simulink model "unicycle_control_template_R2018a"  (R2021a)
settings: Solver=ode23  StartTime=0.0  StopTime=100  RelTol=1e-5
PreLoadFcn:
  | % initialize variables
  | initializeUnicycleModel;
undefined symbols (not defined in the file or in its folder): unicycle
settings Model: Creator=beniamino  LastModifiedBy=pasqu
settings SolverCC: ZeroCrossAlgorithm=Adaptive  AlgebraicLoopSolver=TrustRegion
settings DataIOCC: InitialState=cartesianInitialStates  SaveFormat=StructureWithTime  SaveOutput=off  SignalLogging=off  DSMLogging=off  SaveTime=off  ReturnWorkspaceOutputs=off
settings DebuggingCC: IgnoredZcDiagnostic=none  ArithmeticOperatorsInVariantConditions=warning
settings SFSimCC: CustomCodeUndefinedFunction=UseInterfaceOnly

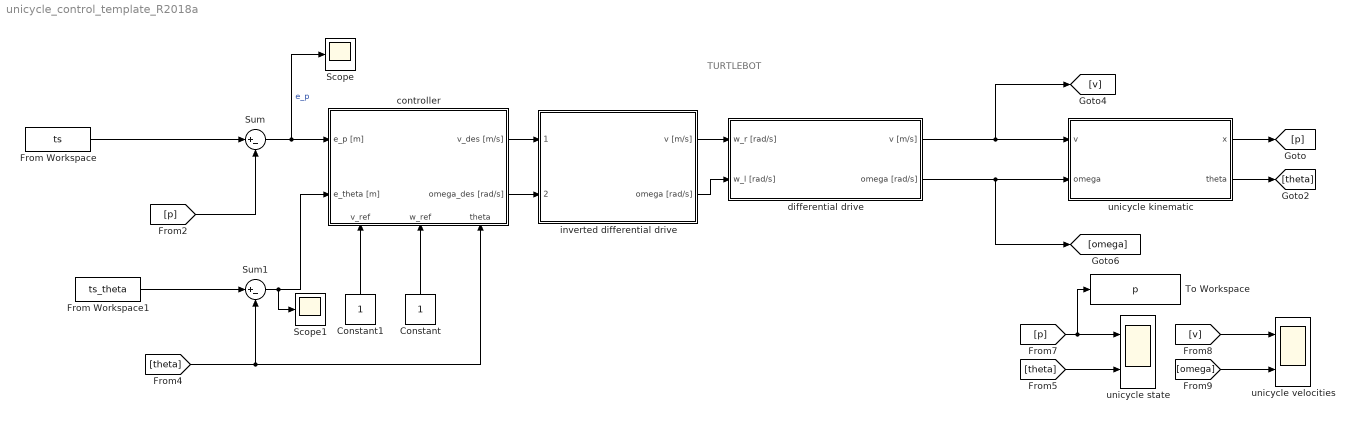
== system unicycle_control_template_R2018a ==
  note: TURTLEBOT
  Constant : Constant
  Constant1 : Constant
  From Workspace : FromWorkspace  VariableName=ts  OutputAfterFinalValue=Holding final value
  From Workspace1 : FromWorkspace  VariableName=ts_theta  OutputAfterFinalValue=Holding final value
  Scope : Scope
  Scope1 : Scope
  Sum : Sum  Inputs=|+-
  Sum1 : Sum  Inputs=|+-
  To Workspace : ToWorkspace  VariableName=p  SaveFormat=Structure With Time  SampleTime=-1
  controller : Subsystem
      settings: PortSchema="{\"entries\":[{\"content\":{\"sides\":[{\"content\":{\"connectorIds\":[\"In1\",\"In2\"]},\"type\":\"ConnectorPlacement.EquallySpacedRectSide\",\"uuid\":\"3f4c2626-0e3e-4d8a-88ac-bb46b09b9e2c\"},{\"content\":{\"connectorIds\":[\"Out1\",\"Out2\"],\"side\":\"RIGHT\"},\"type\":\"ConnectorPlacement.EquallySpacedRectSide\",\"uuid\":\"0c477789-f901-42f2-a0ef-9ff1b1969988\"},{\"content\":{\"connectorIds\":[],\"side\":\"TOP\"},\"type\":\"ConnectorPlacement.EquallySpacedRectSide\",\"uuid\":\"69e4ed00-4175-4f37-9b31-402b95ddf552\"},{\"content\":{\"connectorIds\":[\"In3\",\"In4\",\"In5\"],\"side\":\"BOTTOM\"},\"type\":\"ConnectorPlacement.EquallySpacedRectSide\",\"uuid\":\"a1ef363e-9028-443b-8101-02f6620da377\"}]},\"type\":\"ConnectorPlacement.EquallySpacedConnector\",\"uuid\":\"690776d4-6ae0-4268-9a2b-8a393afd3f2b\"}],\"packageUris\":[\"http://schema.mathworks.com/mf0/Connector/R2020b\"],\"version\":\"1.0\"}"
  differential drive : Subsystem  mask(Differential drive for a unicycle){r=unicycle.diffDrive.r, d=unicycle.diffDrive.d, wheelDyEn=on, Tc=unicycle.diffDrive.Td, wheelsSpeedUpperLimit=unicycle.diffDrive.omegaWheelMax, wheelsSpeedLowerLimit=unicycle.diffDrive.omegaWheelMin}
      mask prompts: r "wheel radius"; d "interaxis lenght"; wheelDyEn "l.p.f. enable"; Tc "time constant [s]"; wheelsSpeedUpperLimit "max wheel speed  [rad/s]"; wheelsSpeedLowerLimit "min wheel speed [rad/s]"
      mask help:
      | Model of a differential drive.
      | It takes as input the derired wheel velocities and converts them to the corresponding driving velocity and stearing velocity.
      | Wheels dynamics can be taken into accont, along with output saturation.
      mask Help:
      | author: Beniamino Pozzan
      | email: beniamino.pozzan@phd.unipd.it
      mask Callback wheelDyEn:
      | % get the enable parameter
      | wheelDyEnStatus = get_param(gcb,'wheelDyEn');
      | enableStatus = get_param(gcb,'MaskEnables');
      | % if it is true, make Tc enabled
      | if strcmp(wheelDyEnStatus,'on')
      |     enableStatus{4}='on';
      | else
      |     enableStatus{4}='off';
      | end
      | set_param(gcb,'MaskEnables',enableStatus)
      mask TypeOptions wheelsSpeedUpperLimit: w_l saturator/UpperLimit | w_r saturator/UpperLimit
      mask TypeOptions wheelsSpeedLowerLimit: w_l saturator/LowerLimit | w_r saturator/LowerLimit
      mask DialogControl wheelDy Prompt: wheel dynamics
  inverted differential drive : Subsystem  mask(Inverted Differential drive for a unicycle){r=unicycle.diffDrive.r, d=unicycle.diffDrive.d}
      mask prompts: r "wheel radius"; d "interaxis lenght"
      mask help:
      | Inverted differential drive for a unicycle.
      | Provided the desired driving and stearing velocities, it computes the corresponding wheel velocities.
  unicycle kinematic : Subsystem  mask(Unicycle Kinematic Model){x0=unicycle.ic.x, y0=unicycle.ic.y, theta0=unicycle.ic.theta}
      mask prompts: x0 "x_0"; y0 "y_0"; theta0 "theta_0"
      mask help: kinematic model of a unicyle.
  unicycle state : Scope  NumInputPorts=2
  unicycle velocities : Scope  NumInputPorts=2
  wires:
  differential drive/1(v [m/s]) -> [v], unicycle kinematic/1(v)
  differential drive/2(omega [rad/s]) -> [omega], unicycle kinematic/2(omega)
  unicycle kinematic/1(x) -> [p]
  unicycle kinematic/2(theta) -> [theta]
  [p] -> Sum/2
  [theta] -> unicycle state/2
  [p] -> To Workspace/1, unicycle state/1
  [v] -> unicycle velocities/1
  [omega] -> unicycle velocities/2
  [theta] -> controller/5(theta), Sum1/2
  Sum1/1 -> Scope1/1, controller/2(e_theta [m])
  Sum/1 -> Scope/1, controller/1(e_p [m])  "e_p"
  Constant/1 -> controller/4(w_ref)
  Constant1/1 -> controller/3(v_ref)
  controller/1(v_des [m/s]) -> inverted differential drive/1(1)
  controller/2(omega_des [rad/s]) -> inverted differential drive/2(2)
  inverted differential drive/2(omega [rad/s]) -> differential drive/2(w_l [rad/s])
  inverted differential drive/1(v [m/s]) -> differential drive/1(w_r [rad/s])
  From Workspace/1 -> Sum/1
  From Workspace1/1 -> Sum1/1

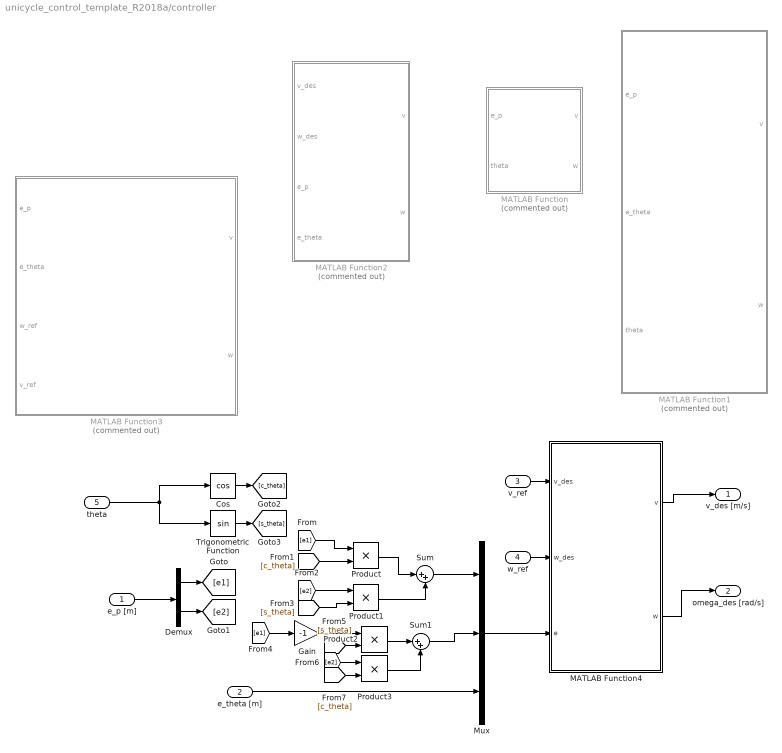
== system unicycle_control_template_R2018a/controller ==
  e_p [m] : Inport
  e_theta [m] : Inport  Port=2
  v_ref : Inport  Port=3
  w_ref : Inport  Port=4
  theta : Inport  Port=5
  Cos : Trigonometry  Operator=cos
  Demux : Demux  Outputs=2
  Gain : Gain  Gain=-1
  MATLAB Function : MATLAB Function  Commented=on  TreatAsAtomicUnit=on
  MATLAB Function1 : MATLAB Function  Commented=on  TreatAsAtomicUnit=on
  MATLAB Function2 : MATLAB Function  Commented=on  TreatAsAtomicUnit=on
  MATLAB Function3 : MATLAB Function  Commented=on  TreatAsAtomicUnit=on
  MATLAB Function4 : MATLAB Function  TreatAsAtomicUnit=on
  Mux : Mux  Inputs=3
  Product{,1..3} (4 alike) : Product
  Sum : Sum  Inputs=|++
  Sum1 : Sum  Inputs=|++
  Trigonometric Function : Trigonometry
  v_des [m/s] : Outport
  omega_des [rad/s] : Outport  Port=2
  wires:
  MATLAB Function4/2(w) -> omega_des [rad/s]/1
  MATLAB Function4/1(v) -> v_des [m/s]/1
  w_ref/1 -> MATLAB Function4/2(w_des)
  v_ref/1 -> MATLAB Function4/1(v_des)
  e_p [m]/1 -> Demux/1
  e_theta [m]/1 -> Mux/3
  Sum1/1 -> Mux/2
  Sum/1 -> Mux/1
  Mux/1 -> MATLAB Function4/3(e)
  theta/1 -> Trigonometric Function/1, Cos/1
  Product/1 -> Sum/1
  Product1/1 -> Sum/2
  Product2/1 -> Sum1/1
  Product3/1 -> Sum1/2
  Demux/1 -> [e1]
  Demux/2 -> [e2]
  Cos/1 -> [c_theta]
  Trigonometric Function/1 -> [s_theta]
  [e1] -> Product/1
  [c_theta] -> Product/2
  [e2] -> Product1/1
  [s_theta] -> Product1/2
  [e1] -> Gain/1
  Gain/1 -> Product2/1
  [s_theta] -> Product2/2
  [e2] -> Product3/1
  [c_theta] -> Product3/2

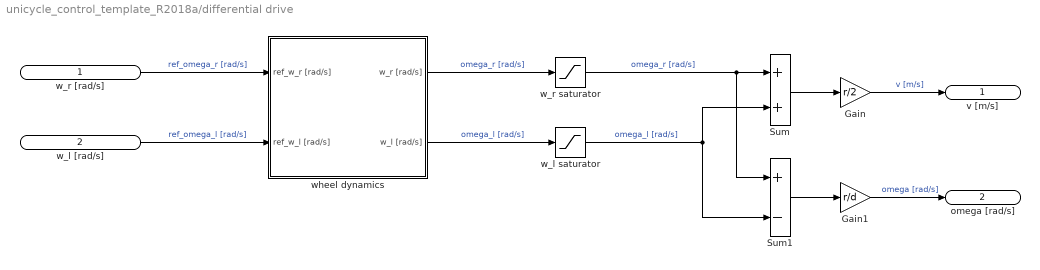
== system unicycle_control_template_R2018a/differential drive ==
  w_r [rad/s] : Inport  Unit=rad/s
  w_l [rad/s] : Inport  Port=2  Unit=rad/s
  Gain : Gain  Gain=r/2
  Gain1 : Gain  Gain=r/d
  Sum : Sum
  Sum1 : Sum  Inputs=+-
  w_l saturator : Saturate  UpperLimit=wheelsSpeedUpperLimit  LowerLimit=wheelsSpeedLowerLimit
  w_r saturator : Saturate  UpperLimit=wheelsSpeedUpperLimit  LowerLimit=wheelsSpeedLowerLimit
  wheel dynamics : Subsystem  Variant=on
  v [m/s] : Outport  Unit=m/s
  omega [rad/s] : Outport  Port=2  Unit=rad/s
  wires:
  w_l saturator/1 -> Sum1/2, Sum/2  "omega_l [rad/s]"
  w_r saturator/1 -> Sum1/1, Sum/1  "omega_r [rad/s]"
  Gain1/1 -> omega [rad/s]/1  "omega [rad/s]"
  Sum1/1 -> Gain1/1
  Gain/1 -> v [m/s]/1  "v [m/s]"
  Sum/1 -> Gain/1
  w_r [rad/s]/1 -> wheel dynamics/1(ref_w_r [rad/s])  "ref_omega_r [rad/s]"
  w_l [rad/s]/1 -> wheel dynamics/2(ref_w_l [rad/s])  "ref_omega_l [rad/s]"
  wheel dynamics/1(w_r [rad/s]) -> w_r saturator/1  "omega_r [rad/s]"
  wheel dynamics/2(w_l [rad/s]) -> w_l saturator/1  "omega_l [rad/s]"

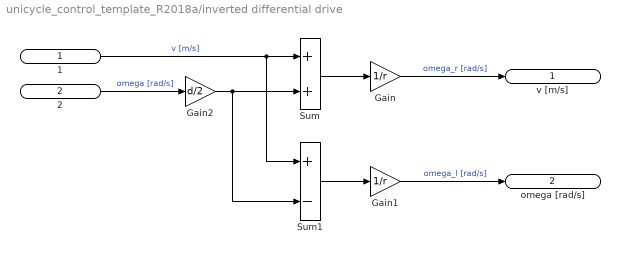
== system unicycle_control_template_R2018a/inverted differential drive ==
  1 : Inport  Unit=m/s
  2 : Inport  Port=2  Unit=rad/s
  Gain : Gain  Gain=1/r
  Gain1 : Gain  Gain=1/r
  Gain2 : Gain  Gain=d/2
  Sum : Sum
  Sum1 : Sum  Inputs=+-
  v [m/s] : Outport  Unit=rad/s
  omega [rad/s] : Outport  Port=2  Unit=rad/s
  wires:
  Gain2/1 -> Sum1/2, Sum/2
  Sum/1 -> Gain/1
  Gain/1 -> v [m/s]/1  "omega_r [rad/s]"
  Sum1/1 -> Gain1/1
  Gain1/1 -> omega [rad/s]/1  "omega_l [rad/s]"
  1/1 -> Sum1/1, Sum/1  "v [m/s]"
  2/1 -> Gain2/1  "omega [rad/s]"

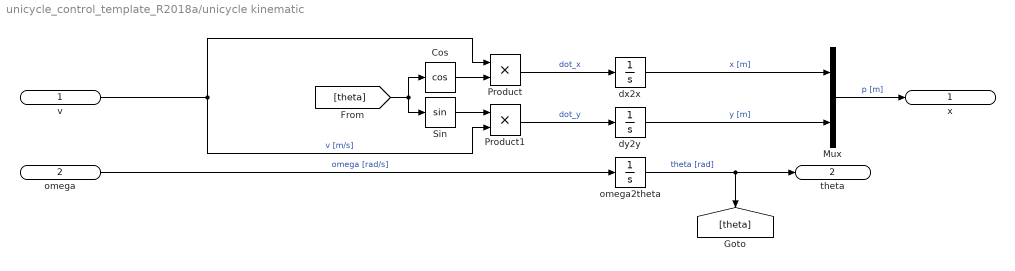
== system unicycle_control_template_R2018a/unicycle kinematic ==
  v : Inport  PortDimensions=1
  omega : Inport  Port=2  PortDimensions=1
  Cos : Trigonometry  Operator=cos
  Mux : Mux  Inputs=2
  Product : Product
  Product1 : Product
  Sin : Trigonometry
  dx2x : Integrator  InitialCondition=x0  ContinuousStateAttributes='pos_x'
  dy2y : Integrator  InitialCondition=y0  ContinuousStateAttributes='pos_y'
  omega2theta : Integrator  InitialCondition=theta0  ContinuousStateAttributes='theta'
  x : Outport  PortDimensions=2
  theta : Outport  Port=2  PortDimensions=1
  wires:
  Product1/1 -> dy2y/1  "dot_y"
  [theta] -> Sin/1, Cos/1
  v/1 -> Product/1, Product1/2  "v [m/s]"
  omega2theta/1 -> [theta], theta/1  "theta [rad]"
  omega/1 -> omega2theta/1  "omega [rad/s]"
  dy2y/1 -> Mux/2  "y [m]"
  Cos/1 -> Product/2
  dx2x/1 -> Mux/1  "x [m]"
  Sin/1 -> Product1/1
  Product/1 -> dx2x/1  "dot_x"
  Mux/1 -> x/1  "p [m]"

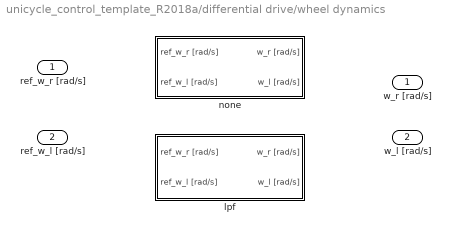
== system unicycle_control_template_R2018a/differential drive/wheel dynamics ==
  ref_w_r [rad/s] : Inport
  ref_w_l [rad/s] : Inport  Port=2
  lpf : Subsystem  VariantControl=wheelDyEn==true
  none : Subsystem  VariantControl=wheelDyEn==false
  w_r [rad/s] : Outport
  w_l [rad/s] : Outport  Port=2

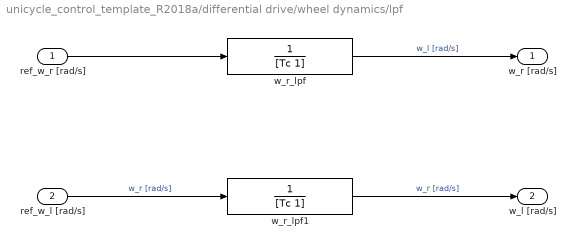
== system unicycle_control_template_R2018a/differential drive/wheel dynamics/lpf ==
  ref_w_r [rad/s] : Inport
  ref_w_l [rad/s] : Inport  Port=2
  w_r_lpf : TransferFcn  Denominator=[Tc 1]  ContinuousStateAttributes='w_r_lpf'
  w_r_lpf1 : TransferFcn  Denominator=[Tc 1]  ContinuousStateAttributes='w_r_lpf'
  w_r [rad/s] : Outport
  w_l [rad/s] : Outport  Port=2
  wires:
  ref_w_r [rad/s]/1 -> w_r_lpf/1
  w_r_lpf1/1 -> w_l [rad/s]/1  "w_r [rad/s]"
  w_r_lpf/1 -> w_r [rad/s]/1  "w_l [rad/s]"
  ref_w_l [rad/s]/1 -> w_r_lpf1/1  "w_r [rad/s]"

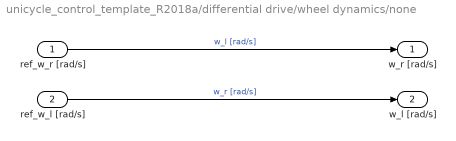
== system unicycle_control_template_R2018a/differential drive/wheel dynamics/none ==
  ref_w_r [rad/s] : Inport
  ref_w_l [rad/s] : Inport  Port=2
  w_r [rad/s] : Outport
  w_l [rad/s] : Outport  Port=2
  wires:
  ref_w_r [rad/s]/1 -> w_r [rad/s]/1  "w_l [rad/s]"
  ref_w_l [rad/s]/1 -> w_l [rad/s]/1  "w_r [rad/s]"

== matlab function unicycle_control_template_R2018a/controller/MATLAB Function1 ==
  data: e_p input; v output; e_theta input; theta input; w output
function [v,w] = postureController(e_p,e_theta,theta)
rho=norm(e_p);
gamma=atan2(e_p(2),e_p(1))-theta;
delta=gamma-e_theta;
Kv=1;
Kw=1;
Kd=5;
v=Kv*rho*cos(gamma);
w=Kw*gamma+Kv*((sin(gamma)*cos(gamma))/gamma)*(gamma+Kd*delta);

== matlab function unicycle_control_template_R2018a/controller/MATLAB Function ==
  data: e_p input; v output; theta input; w output
function [v,w] = positionController(e_p,theta)
Kv=2;
Kw=0.1;
v=Kv*(e_p(1)*cos(theta)+e_p(2)*sin(theta));
w=Kw*(atan2(e_p(2),e_p(1))-theta);

== matlab function unicycle_control_template_R2018a/controller/MATLAB Function2 ==
  data: v_des input; v output; w output; w_des input; e_p input; e_theta input
function [v,w] = trajectoryController(v_des,w_des,e_p,e_theta)
xi=0.2;
a=10;
k1=2*xi*a;
k2=(a^2-w_des^2)/v_des;
k3=k1;
v=norm(v_des)*cos(e_theta)-k1*e_p(1);
w=w_des-k2*e_p(2)-k3*e_theta;

== matlab function unicycle_control_template_R2018a/controller/MATLAB Function3 ==
  data: e_p input; v output; e_theta input; w_ref input; v_ref input; w output
function [v,w]= nonlinearTrackingController(e_p,e_theta,w_ref,v_ref)
k2=1;
k1=w_ref*(2+sin(norm(v_ref)));
k3=w_ref*(2+cos(norm(v_ref)));
v=-k1*e_p(1);
w=-k2*norm(v_ref)*(sin(e_theta)/e_theta)*e_p(2)-k3*e_theta;

== matlab function unicycle_control_template_R2018a/controller/MATLAB Function4 ==
  data: v_des input; v output; w output; w_des input; e input
function [v,w] = trajectoryController(v_des,w_des,e)
xi=0.5;
a=10000;
k1=2*xi*a;
k2=(a^2-w_des^2)/v_des;
k3=k1;
v=v_des*cos(e(3))+k1*e(1);
w=w_des+k2*e(2)+k3*e(3);
